simulink model "Ref_park_clarke"  (R2022b)
settings: Solver=ode23tb  StartTime=0.0  StopTime=0.1  MaxStep=1e-6  RelTol=1e-3
values from neighbouring files (symbols this model uses):
  Lf = 100e-3    (= 0.1)    [RL_parameters.m]
  Lm = 80e-3    (= 0.08)    [RL_parameters.m]
  R = 2    [RL_parameters.m]
libraries: spsabctodq0Lib x1
settings Model: Creator=benve  LastModifiedBy=benve

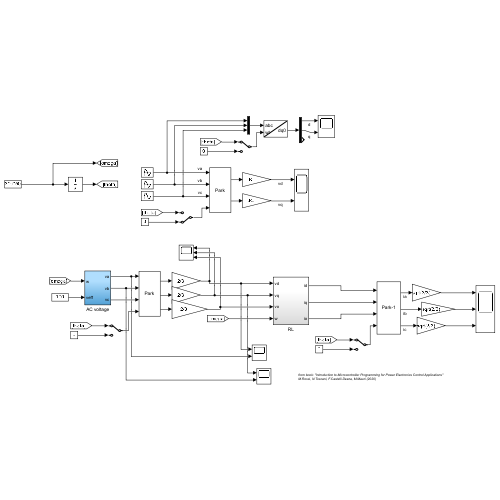
[thumbnail: Simulink's stored preview of the top-level diagram]
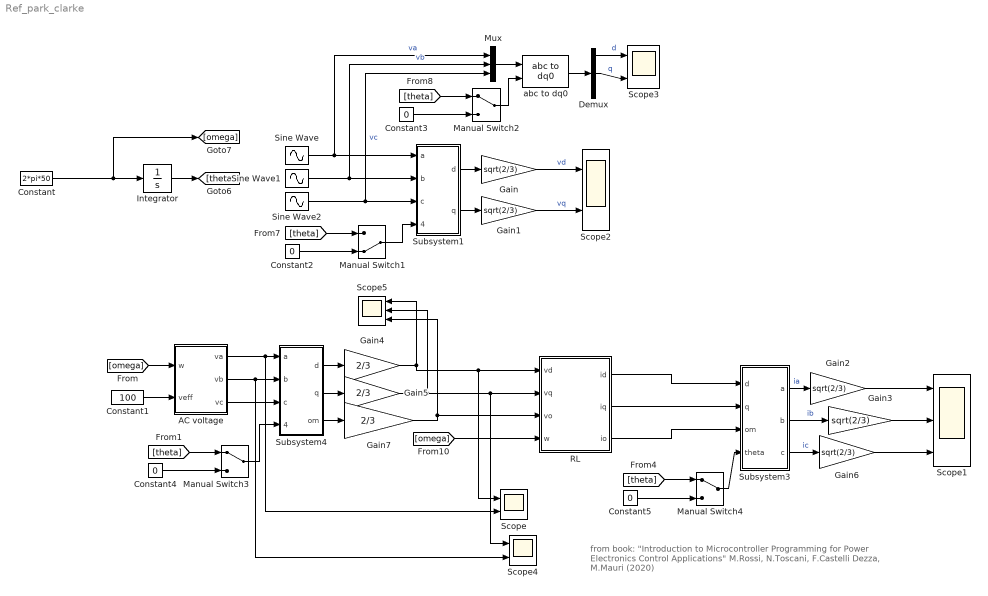
== system Ref_park_clarke ==
  note: from book: "Introduction to Microcontroller Programming for Power Electronics Control Applications"
      | M.Rossi, N.Toscani, F.Castelli Dezza, M.Mauri (2020)
  AC voltage : Subsystem
  Constant : Constant  Value=2*pi*50
  Constant1 : Constant  Value=100
  Constant{2..5} (4 alike) : Constant  Value=0
  Demux : Demux  Outputs=3
  Gain{,1..3,6} (5 alike) : Gain  Gain=sqrt(2/3)
  Gain4 : Gain  Gain=2/3
  Gain5 : Gain  Gain=2/3
  Gain7 : Gain  Gain=2/3
  Integrator : Integrator
  Manual Switch1 : ManualSwitch  CurrentSetting=0
  Manual Switch2 : ManualSwitch
  Manual Switch3 : ManualSwitch
  Manual Switch4 : ManualSwitch
  Mux : Mux  Inputs=3
  RL : Subsystem
  Scope{,2..4} (4 alike) : Scope  NumInputPorts=2
  Scope1 : Scope  NumInputPorts=3
  Scope5 : Scope  NumInputPorts=3
  Sine Wave : Sin  Amplitude=100*sqrt(2)  Frequency=2*pi*50  SampleTime=0
  Sine Wave1 : Sin  Amplitude=100*sqrt(2)  Frequency=2*pi*50  Phase=-2*pi/3  SampleTime=0
  Sine Wave2 : Sin  Amplitude=100*sqrt(2)  Frequency=2*pi*50  Phase=-4*pi/3  SampleTime=0
  Subsystem1 : Subsystem
      mask Display: disp('Park')
  Subsystem3 : Subsystem
      mask Display: disp('Park-1')
  Subsystem4 : Subsystem
      mask Display: disp('Park')
  abc to dq0 : spsabctodq0Lib/abc to dq0  Alignment=Aligned with phase A axis
  wires:
  RL/2(iq) -> Subsystem3/2(q)
  RL/1(id) -> Subsystem3/1(d)
  RL/3(io) -> Subsystem3/3(om)
  Manual Switch1/1 -> Subsystem1/4(theta)
  Subsystem3/2(b) -> Gain3/1  "ib"
  Manual Switch2/1 -> abc to dq0/2
  Gain7/1 -> Scope5/3, RL/3(vo)
  [theta] -> Manual Switch4/1
  Gain6/1 -> Scope1/3
  [theta] -> Manual Switch3/1
  Demux/1 -> Scope3/1  "d"
  Subsystem4/3(om) -> Gain7/1
  [omega] -> AC voltage/1(w)
  AC voltage/3(vc) -> Subsystem4/3(c)
  Constant5/1 -> Manual Switch4/2
  Subsystem3/3(c) -> Gain6/1  "ic"
  Gain3/1 -> Scope1/2
  Constant4/1 -> Manual Switch3/2
  [omega] -> RL/4(w)
  Sine Wave2/1 -> Mux/3, Subsystem1/3(c)  "vc"
  Subsystem3/1(a) -> Gain2/1  "ia"
  abc to dq0/1 -> Demux/1
  Subsystem4/1(d) -> Gain4/1
  AC voltage/1(va) -> Scope/2, Subsystem4/1(a)
  [theta] -> Manual Switch1/1
  [theta] -> Manual Switch2/1
  Constant3/1 -> Manual Switch2/2
  Subsystem1/1(d) -> Gain/1
  Gain/1 -> Scope2/1  "vd"
  Demux/2 -> Scope3/2  "q"
  Subsystem4/2(q) -> Gain5/1
  Constant1/1 -> AC voltage/2(veff)
  Gain2/1 -> Scope1/1
  Constant2/1 -> Manual Switch1/2
  AC voltage/2(vb) -> Scope4/2, Subsystem4/2(b)
  Gain1/1 -> Scope2/2  "vq"
  Subsystem1/2(q) -> Gain1/1
  Gain4/1 -> Scope5/1, Scope/1, RL/1(vd)
  Mux/1 -> abc to dq0/1
  Sine Wave1/1 -> Mux/2, Subsystem1/2(b)  "vb"
  Manual Switch3/1 -> Subsystem4/4(theta)
  Sine Wave/1 -> Mux/1, Subsystem1/1(a)  "va"
  Gain5/1 -> Scope5/2, Scope4/1, RL/2(vq)
  Integrator/1 -> [theta]
  Constant/1 -> [omega], Integrator/1
  Manual Switch4/1 -> Subsystem3/4(theta)

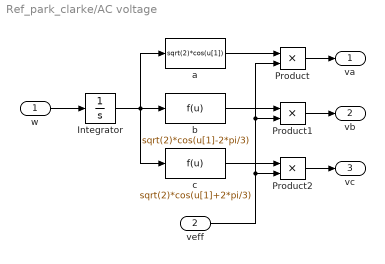
== system Ref_park_clarke/AC voltage ==
  w : Inport
  veff : Inport  Port=2
  Integrator : Integrator
  Product : Product  InputSameDT=on  RndMeth=Zero  SaturateOnIntegerOverflow=on  OutDataTypeStr=Inherit: Same as first input
  Product1 : Product  InputSameDT=on  RndMeth=Zero  SaturateOnIntegerOverflow=on  OutDataTypeStr=Inherit: Same as first input
  Product2 : Product  InputSameDT=on  RndMeth=Zero  SaturateOnIntegerOverflow=on  OutDataTypeStr=Inherit: Same as first input
  "a " : Fcn  Expr=sqrt(2)*cos(u[1])
  "b " : Fcn  Expr=sqrt(2)*cos(u[1]-2*pi/3)
  "c " : Fcn  Expr=sqrt(2)*cos(u[1]+2*pi/3)
  va : Outport  VectorParamsAs1DForOutWhenUnconnected=off
  vb : Outport  Port=2  VectorParamsAs1DForOutWhenUnconnected=off
  vc : Outport  Port=3  VectorParamsAs1DForOutWhenUnconnected=off
  wires:
  Integrator/1 -> "c "/1, "a "/1, "b "/1
  w/1 -> Integrator/1
  "a "/1 -> Product/1
  veff/1 -> Product2/2, Product1/2, Product/2
  Product/1 -> va/1
  "b "/1 -> Product1/1
  "c "/1 -> Product2/1
  Product1/1 -> vb/1
  Product2/1 -> vc/1

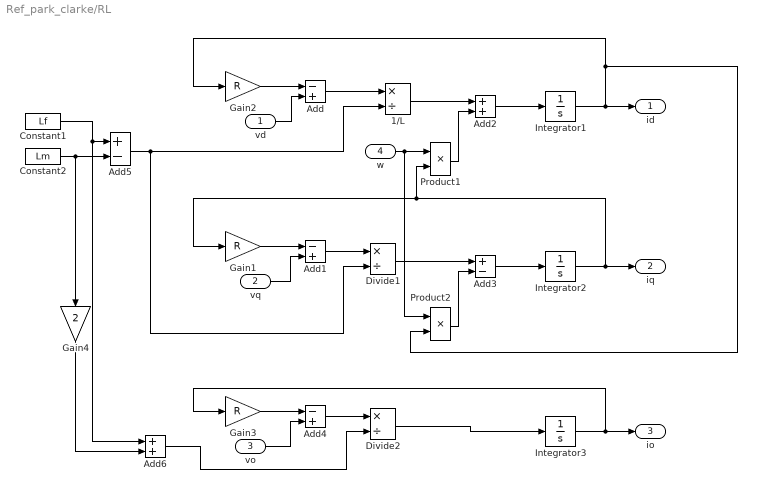
== system Ref_park_clarke/RL ==
  vd : Inport
  vq : Inport  Port=2
  vo : Inport  Port=3
  w : Inport  Port=4
  1/L : Product  Inputs=*/
  Add : Sum  Inputs=-+
  Add1 : Sum  Inputs=-+
  Add2 : Sum
  Add3 : Sum  Inputs=+-
  Add4 : Sum  Inputs=-+
  Add5 : Sum  Inputs=+-
  Add6 : Sum
  Constant1 : Constant  Value=Lf
  Constant2 : Constant  Value=Lm
  Divide1 : Product  Inputs=*/
  Divide2 : Product  Inputs=*/
  Gain1 : Gain  Gain=R
  Gain2 : Gain  Gain=R
  Gain3 : Gain  Gain=R
  Gain4 : Gain  Gain=2
  Integrator1 : Integrator
  Integrator2 : Integrator
  Integrator3 : Integrator
  Product1 : Product
  Product2 : Product
  id : Outport  VectorParamsAs1DForOutWhenUnconnected=off
  iq : Outport  Port=2  VectorParamsAs1DForOutWhenUnconnected=off
  io : Outport  Port=3  VectorParamsAs1DForOutWhenUnconnected=off
  wires:
  Gain2/1 -> Add/1
  vd/1 -> Add/2
  Add/1 -> 1/L/1
  1/L/1 -> Add2/1
  Add2/1 -> Integrator1/1
  Integrator1/1 -> Product2/2, Gain2/1, id/1
  Product1/1 -> Add2/2
  Gain1/1 -> Add1/1
  vq/1 -> Add1/2
  Add1/1 -> Divide1/1
  Divide1/1 -> Add3/1
  Add3/1 -> Integrator2/1
  Integrator2/1 -> Product1/2, Gain1/1, iq/1
  Product2/1 -> Add3/2
  w/1 -> Product1/1, Product2/1
  Gain3/1 -> Add4/1
  vo/1 -> Add4/2
  Add4/1 -> Divide2/1
  Divide2/1 -> Integrator3/1
  Integrator3/1 -> Gain3/1, io/1
  Constant1/1 -> Add6/1, Add5/1
  Constant2/1 -> Add5/2, Gain4/1
  Add5/1 -> Divide1/2, 1/L/2
  Gain4/1 -> Add6/2
  Add6/1 -> Divide2/2

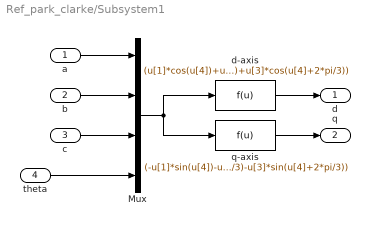
== system Ref_park_clarke/Subsystem1 ==
  a : Inport
  b : Inport  Port=2
  c : Inport  Port=3
  theta : Inport  Port=4
  Mux : Mux
  d-axis : Fcn  Expr=(u[1]*cos(u[4])+u[2]*cos(u[4]-2*pi/3)+u[3]*cos(u[4]+2*pi/3))
  q-axis : Fcn  Expr=(-u[1]*sin(u[4])-u[2]*sin(u[4]-2*pi/3)-u[3]*sin(u[4]+2*pi/3))
  d : Outport  VectorParamsAs1DForOutWhenUnconnected=off
  q : Outport  Port=2  VectorParamsAs1DForOutWhenUnconnected=off
  wires:
  b/1 -> Mux/2
  a/1 -> Mux/1
  q-axis/1 -> q/1
  d-axis/1 -> d/1
  c/1 -> Mux/3
  theta/1 -> Mux/4
  Mux/1 -> q-axis/1, d-axis/1

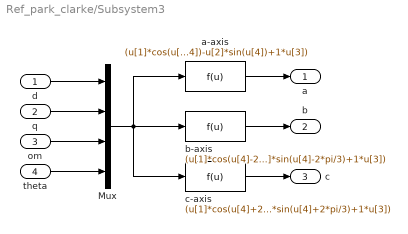
== system Ref_park_clarke/Subsystem3 ==
  d : Inport
  q : Inport  Port=2
  om : Inport  Port=3
  theta : Inport  Port=4
  Mux : Mux
  a-axis : Fcn  Expr=(u[1]*cos(u[4])-u[2]*sin(u[4])+1*u[3])
  b-axis : Fcn  Expr=(u[1]*cos(u[4]-2*pi/3)-u[2]*sin(u[4]-2*pi/3)+1*u[3])
  c-axis : Fcn  Expr=(u[1]*cos(u[4]+2*pi/3)-u[2]*sin(u[4]+2*pi/3)+1*u[3])
  a : Outport  VectorParamsAs1DForOutWhenUnconnected=off
  b : Outport  Port=2  VectorParamsAs1DForOutWhenUnconnected=off
  c : Outport  Port=3  VectorParamsAs1DForOutWhenUnconnected=off
  wires:
  q/1 -> Mux/2
  d/1 -> Mux/1
  b-axis/1 -> b/1
  a-axis/1 -> a/1
  theta/1 -> Mux/4
  Mux/1 -> a-axis/1, c-axis/1, b-axis/1
  c-axis/1 -> c/1
  om/1 -> Mux/3

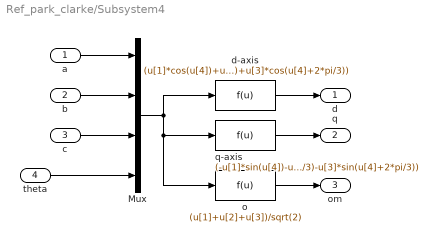
== system Ref_park_clarke/Subsystem4 ==
  a : Inport
  b : Inport  Port=2
  c : Inport  Port=3
  theta : Inport  Port=4
  Mux : Mux
  d-axis : Fcn  Expr=(u[1]*cos(u[4])+u[2]*cos(u[4]-2*pi/3)+u[3]*cos(u[4]+2*pi/3))
  o : Fcn  Expr=(u[1]+u[2]+u[3])/sqrt(2)
  q-axis : Fcn  Expr=(-u[1]*sin(u[4])-u[2]*sin(u[4]-2*pi/3)-u[3]*sin(u[4]+2*pi/3))
  d : Outport  VectorParamsAs1DForOutWhenUnconnected=off
  q : Outport  Port=2  VectorParamsAs1DForOutWhenUnconnected=off
  om : Outport  Port=3  VectorParamsAs1DForOutWhenUnconnected=off
  wires:
  b/1 -> Mux/2
  a/1 -> Mux/1
  q-axis/1 -> q/1
  d-axis/1 -> d/1
  c/1 -> Mux/3
  theta/1 -> Mux/4
  Mux/1 -> o/1, q-axis/1, d-axis/1
  o/1 -> om/1
